simulink library "carnot"  (R2013b)
settings: Solver=ode45  StartTime=0.0  StopTime=10.0  RelTol=1e-3
undefined symbols (not defined in the file or in its folder): A, acol, Ahabit, Awin, Azimuth_Angle, AziWin, B, C, c1, c4, capc, caph, CarnotCallbacks_Density, CarnotCallbacks_Enthalpy, CarnotCallbacks_Enthalpy2Temperature, CarnotCallbacks_Entropy, CarnotCallbacks_Evaporation_Enthalpy, CarnotCallbacks_GlobalMessageLevel, CarnotCallbacks_Grashof, CarnotCallbacks_Heat_Capacity, CarnotCallbacks_Kinematic_Viscosity, CarnotCallbacks_Prandtl, CarnotCallbacks_Saturation_Property, CarnotCallbacks_Saturation_Temperature, CarnotCallbacks_Saturation_Value_Water, CarnotCallbacks_Specific_Volume, CarnotCallbacks_Thermal_Conductivity, CarnotCallbacks_Vapour_Content, CarnotCallbacks_Vapour_Pressure, con, cond, d, Dd, density, dfin, dia, DiameterLastPiece, DPConstant, dpipe, DPLinear, DPQuadratic, emission_out, fluid, FluidMix, FluidType, FPC, frame, g, GeodeticHeight, Gwin, heat_capacity, hgt, HP, Hroom, ID, inlet, K, l, lin, lpipe ... (+29)
undefined symbols (not defined in the file): c2, c3, c5, c6, cwall, dactive, height, mc, mID, rho, tau, UAneighbour, UAwall, uloss
libraries: carnot x333, simulink x25, simulink_extras x7
(part 5 of 16)

== system carnot/Basic/Weather_and_Sun ==
  Cloudage : Subsystem  mask(cloud index){latitude=51, longitude=-7, longitude0=-30, skytype=high mountain}
      mask prompts: latitude "Latitude [-90;90], north positive"; longitude "Longitude  [-180;180], west positive"; longitude0 "reference longitude (timezone)"; skytype "Sky Type"
      mask help:
      | Calculates the cloud index. The cloud index is the fraction of the sky covered by clouds in [0, 1/8, 2/8, 3/8, ..., 7/8, 1].
      |
      | INPUT VECTOR:
      |  time    : real time or simulation time [s]
      |  Iglob   : global radiation on horizontal surface (W/m²)
      |
      | OUTPUT VECTOR:
      |  cloud  : cloudindex [0;1]
      mask Help: web(fullfile(path_carnot('help'),'Cloudage.html'),'-helpbrowser')
      mask TypeOptions skytype: high mountain | lowland | urban region | industrial zone
  Radiation_Divison : Subsystem  mask(Radiation Division){latitude=51, longitude=-7, longitude0=-30}
      mask prompts: latitude "Latitude [-90;90], north positive"; longitude "Longitude  [-180;180], west positive"; longitude0 "reference longitude (timezone)"
      mask help:
      | Calculates the direct and diffusive radiation on the horizontal surface as parts of the global radiation.
      |
      | INPUT VECTOR:
      |   time      : real time or simulation time  [s]
      |   Iglob     : global radiation on horizontal surface (W/m²)
      |
      | OUTPUT VECTORS:
      |   Idir           : direct radiation (W/m²)
      |   Idfu          : diffusive radiation (W/m²)
      |   SunAngle
      |   Zenith
      |   Azimuth
      mask Help: web(fullfile(path_carnot('help'),'Radiation_Divison.html'),'-helpbrowser')
  Sky_Temperature : Subsystem  mask(Sky Temperature){tskymodel=on}
      mask prompts: tskymodel "Include time correction (cos-term in Berdahl equation)"
      mask help:
      | Calculates the skytemperature. If humidity data is availabe, the model of Berdahl and Martin 1984 for low clouds (1000 m) is used.
      | Without humidity data, the model of Unsworth with corrected parameters of Feist 1994 is chosen.
      | INPUT VECTOR:
      |   tamb : ambient temperature [°C]
      |   hum  : humidity [%]
      |   cloud: index of cloudness [0,1]
      |
      | OUTPUT VECTOR:
      |   tsky : sky temperature [°C]
      |
      | The calculation can also be used in m-files with the skytemperature.m function.
      mask Help: web(fullfile(path_carnot('help'),'Sky_Temperature.html'),'-helpbrowser')
  Solar_Declination_Angle : Subsystem  mask(solar declination angle){}
      mask help:
      | The block calls the function "solar_declination" in the CARNOT Library
      | Carlib where the calculation is effectuated. The function solar_declination
      | may be used in m-files. The carlib function solar_declination is also
      | used by the "solar_declination"-block in CARNOT.
      | The equation was taken from Duffie, Beckmann: Solar Engineering of
      | Thermal Processes, 2006. Orginaly the equation was derived by Spencer
      | (Spencer: Fourier Series Representation of the Position of the Sun,
      |  Search Vol.2(5), page 172 , 1971). The error is below 0.035°.
      mask Help: web(fullfile(path_carnot('help'),'Solar_Declination_Angle.html'),'-helpbrowser')
  Solar_Extraterrestrial_Radiation : Subsystem  mask(solar extraterrestrial radiation){}
      mask help:
      | The block calls the function "extraterrestrial_radiation" in the CARNOT Library
      | Carlib where the calculation is effectuated. The function solar_extraterrestrial
      | may be used in m-files. The carlib function extraterrestrial_radiation is also
      | used by the "solar_extraterrestrial_radiation"-block in CARNOT.
      | The equation was taken from Duffie, Beckmann: Solar Engineering of
      | Thermal Processes, 2006. Orginaly the equation was derived by Spencer
      | (Spencer: Fourier Series Representation of the Position of the Sun,
      |  Search Vol.2(5), page 172 , 1971). The accuracy is +- 0.01 %
      mask Help: web(fullfile(path_carnot('help'),'Solar_Extraterrestrial_Radiation.html'),'-helpbrowser')
  Solar_Hour_Angle : Subsystem  mask(Solar Hour Angle){timezone=-15, longitude=-7}
      mask prompts: timezone "longitude of timezone (GMT = 0, east negative) in degree"; longitude "longitude of location (east negative) in degree"
      mask help:
      | The block calls the function "solar_hour_angle" in the CARNOT Library
      | Carlib where the calculation is effectuated.
      | The equation was taken from Duffie, Beckmann: Solar Engineering of
      | Thermal Processes, 2006.
      mask Help: web(fullfile(path_carnot('help'),'Solar_Hour_Angle.html'),'-helpbrowser')
  Solar_Position : Subsystem  mask(Solar Position){lati=45, longi=0, timezone=0}
      mask prompts: lati "Geographical latitude in degree (North postive)"; longi "Geographical longitude in degree (West postive)"; timezone "Latitude of timezone in degree (West postive)"
      mask help:
      | Calculate the solar postion (Duffie, Beckman: Solar Engineering of Thermal Processes, 2008).
      | Output is:
      mask Help: web(fullfile(path_carnot('help'),'Solar_Position.html'),'-helpbrowser')
      mask Display: disp('sunpos')
  Solar_Time : Subsystem  mask(solar time){timezone=-15, longitude=-7}
      mask prompts: timezone "longitude of timezone (GMT = 0, east negative) in degree"; longitude "longitude of location (east negative) in degree"
      mask help:
      | The block calls the function "solar_time" in the CARNOT Library
      | Carlib where the calculation is effectuated. The function solar_time
      | may be used in m-files as "solartime2legaltime" or "legaltime2solartime".
      | The carlib function solar_time is also used by the "solar_time"-block in CARNOT.
      | The equation was taken from Duffie, Beckmann: Solar Engineering of
      | Thermal Processes, 2006. Orginaly the equation was derived by Spencer
      | (Spencer: Fourier Series Representation of the Position of the Sun,
      |  Search Vol.2(5), page 172 , 1971). The accuracy is +- 0.01 %
      mask Help: web(fullfile(path_carnot('help'),'Solar_Time.html'),'-helpbrowser')
  WDB_Creator : Subsystem  mask(Weather Data Bus Creator){}
      mask help: Create the weather data bus with scalar inputs.
      mask Help: web(fullfile(path_carnot('help'),'WDB_Creator.html'),'-helpbrowser')

== system carnot/Control/Controller_Bang_Bang ==
  Thot : Inport
  Tcold : Inport  Port=2
  Constant : Constant  Value=Tmax
  MinMax : MinMax  Function=max  Inputs=2  SaturateOnIntegerOverflow=on  InputSameDT=on
  Product : Product  OutDataTypeStr=double  SaturateOnIntegerOverflow=on
  Relational Operator : RelationalOperator  Operator=<=  InputSameDT=on
  Relay : Relay  OnSwitchValue=deltaTon  OffSwitchValue=deltaToff
  Sum : Sum  Inputs=-+  SaturateOnIntegerOverflow=on  InputSameDT=on  OutDataTypeStr=Inherit: Same as first input
  control : Outport
  wires:
  Sum/1 -> Relay/1
  Constant/1 -> Relational Operator/2
  Thot/1 -> Sum/2, MinMax/2
  Tcold/1 -> Sum/1, MinMax/1
  MinMax/1 -> Relational Operator/1
  Relay/1 -> Product/1
  Product/1 -> control/1
  Relational Operator/1 -> Product/2

== system carnot/Control/EnergyMeter ==
  note: Shows the power in W and the energy in J gain or loss
      | in a fluid flow (characterised by THB) between the
      | inlet and the outlet of one component.
  THB_out : Inport
  THB_in : Inport  Port=2
  Integrator : Integrator  UpperSaturationLimit=1  LowerSaturationLimit=0
  PowerMeter : carnot/Control/PowerMeter
  energy : Outport
  power : Outport  Port=2
  wires:
  THB_out/1 -> PowerMeter/1
  Integrator/1 -> energy/1
  THB_in/1 -> PowerMeter/2
  PowerMeter/1 -> power/1, Integrator/1

== system carnot/Control/EnergyMeter_HC ==
  note: Shows the power in W and the energy in J gain or loss
      | in a fluid flow (characterised by THV) between the
      | inlet and the outlet of one component.
  THB_out : Inport
  THB_in : Inport  Port=2
  Bus Selector : BusSelector  OutputSignals=Temperature
  Bus Selector1 : BusSelector  OutputSignals=Temperature,MassFlow,Pressure,FluidType,FluidMix
  Heat_Capacity : Reference
  Integrator : Integrator  UpperSaturationLimit=1  LowerSaturationLimit=0
  Integrator1 : Integrator  UpperSaturationLimit=1  LowerSaturationLimit=0
  Product : Product  Inputs=***  SaturateOnIntegerOverflow=on  RndMeth=Zero  InputSameDT=on  OutDataTypeStr=Inherit: Same as first input
  T_ave : Gain  Gain=0.5  SaturateOnIntegerOverflow=on  OutDataTypeStr=Inherit: Same as input  ParamDataTypeStr=Inherit: Same as input
  diff_T : Sum  Inputs=+-  SaturateOnIntegerOverflow=on  InputSameDT=on  OutDataTypeStr=Inherit: Same as first input
  only_negative : Saturate  UpperLimit=0  LowerLimit=-inf
  only_positive : Saturate  UpperLimit=inf  LowerLimit=0
  sum : Sum  SaturateOnIntegerOverflow=on  InputSameDT=on  OutDataTypeStr=Inherit: Same as first input
  heating energy : Outport  InitialOutput=0
  power : Outport  Port=2  InitialOutput=0
  cooling energy : Outport  Port=3  InitialOutput=0
  wires:
  THB_in/1 -> Bus Selector/1
  THB_out/1 -> Bus Selector1/1
  Bus Selector1/1 -> diff_T/1, sum/1  "<Temperature>"
  Bus Selector1/4 -> Heat_Capacity/3  "<FluidType>"
  Bus Selector1/5 -> Heat_Capacity/4  "<FluidMix>"
  Heat_Capacity/1 -> Product/1
  Integrator/1 -> heating energy/1
  Bus Selector1/2 -> Product/2  "<MassFlow>"
  diff_T/1 -> Product/3
  Bus Selector/1 -> diff_T/2, sum/2  "<Temperature>"
  sum/1 -> T_ave/1
  T_ave/1 -> Heat_Capacity/1
  Bus Selector1/3 -> Heat_Capacity/2  "<Pressure>"
  Integrator1/1 -> cooling energy/1
  Product/1 -> power/1, only_negative/1, only_positive/1
  only_negative/1 -> Integrator1/1
  only_positive/1 -> Integrator/1

== system carnot/Control/Massflow_Sensor ==
  THB_in : Inport
  Bus Selector : BusSelector  OutputSignals=MassFlow
  heat capacity : StateSpace  A=-tc  B=tc  D=0  X0=t0
  THB : Outport
  mdot : Outport  Port=2
  wires:
  THB_in/1 -> THB/1, Bus Selector/1
  Bus Selector/1 -> heat capacity/1  "<MassFlow>"
  heat capacity/1 -> mdot/1

== system carnot/Control/Max_Run_Time ==
  In : Inport
  Compare To Zero : simulink/Logic and Bit Operations/Compare To Zero  relop=>  OutDataTypeStr=uint8
  Constant : Constant  Value=-1
  Integrator : Integrator  ExternalReset=rising  InitialCondition=tmaxrun  LimitOutput=on  LowerSaturationLimit=0
  Product : Product  RndMeth=Zero
  Out : Outport
  wires:
  Constant/1 -> Integrator/1
  Integrator/1 -> Compare To Zero/1
  Compare To Zero/1 -> Product/1
  In/1 -> Product/2, Integrator/2
  Product/1 -> Out/1

== system carnot/Control/Min_Run_Time ==
  In : Inport
  Compare To Zero : simulink/Logic and Bit Operations/Compare To Zero  relop=>  OutDataTypeStr=uint8
  Constant : Constant  Value=-1
  Gain : Gain  Gain=mv
  Integrator : Integrator  ExternalReset=rising  InitialCondition=tminrun  LimitOutput=on  LowerSaturationLimit=0
  MinMax : MinMax  Function=max  Inputs=2
  Out : Outport
  wires:
  MinMax/1 -> Out/1
  In/1 -> MinMax/2, Integrator/2
  Compare To Zero/1 -> Gain/1
  Integrator/1 -> Compare To Zero/1
  Constant/1 -> Integrator/1
  Gain/1 -> MinMax/1

== system carnot/Control/Min_Stop_Time ==
  In : Inport
  Compare To Zero : simulink/Logic and Bit Operations/Compare To Zero  relop=<=  OutDataTypeStr=uint8
  Compare To Zero1 : simulink/Logic and Bit Operations/Compare To Zero  relop=<=  OutDataTypeStr=uint8
  Constant : Constant  Value=-1
  Integrator : Integrator  ExternalReset=falling  InitialConditionSource=external  InitialCondition=tminstop  LimitOutput=on  LowerSaturationLimit=0  ShowStatePort=on
  Product : Product  RndMeth=Zero
  Product1 : Product  RndMeth=Zero
  Step : Step  Time=0.1  After=tminstop  SampleTime=0
  Out : Outport
  wires:
  Step/1 -> Integrator/3
  Compare To Zero1/1 -> Product/1
  Integrator/State -> Compare To Zero1/1
  Product/1 -> Integrator/2
  Product1/1 -> Out/1
  In/1 -> Product1/2, Product/2
  Compare To Zero/1 -> Product1/1
  Integrator/1 -> Compare To Zero/1
  Constant/1 -> Integrator/1

== system carnot/Control/PowerMeter ==
  THB_out : Inport
  THB_in : Inport  Port=2
  Bus Selector : BusSelector  OutputSignals=Temperature
  Bus Selector1 : BusSelector  OutputSignals=Temperature,MassFlow,Pressure,FluidType,FluidMix
  Heat_Capacity : carnot/Basic/Material_Properties/Heat_Capacity  VariantControl=CarlibClassic  INPUTARGUMENTS=state variables (classic)  DEBUGLEVEL=DEBUGLEVEL  MAXTOTALWARNINGS=inf  MAXCONSECUTIVEWARNINGS=inf  WRITETOFILE=0  FILENAME='errors.txt'
  Product : Product  Inputs=***  SaturateOnIntegerOverflow=on  InputSameDT=on  OutDataTypeStr=Inherit: Same as first input
  T_ave : Gain  Gain=0.5  SaturateOnIntegerOverflow=on  OutDataTypeStr=Inherit: Same as input  ParamDataTypeStr=Inherit: Same as input
  diff_T : Sum  Inputs=+-  SaturateOnIntegerOverflow=on  InputSameDT=on  OutDataTypeStr=Inherit: Same as first input
  sum : Sum  SaturateOnIntegerOverflow=on  InputSameDT=on  OutDataTypeStr=Inherit: Same as first input
  power : Outport
  wires:
  Bus Selector1/1 -> diff_T/1, sum/1  "<Temperature>"
  Bus Selector1/4 -> Heat_Capacity/3  "<FluidType>"
  Bus Selector1/5 -> Heat_Capacity/4  "<FluidMix>"
  Heat_Capacity/1 -> Product/1
  Product/1 -> power/1
  Bus Selector1/2 -> Product/2  "<MassFlow>"
  diff_T/1 -> Product/3
  THB_in/1 -> Bus Selector/1
  Bus Selector/1 -> diff_T/2, sum/2  "<Temperature>"
  sum/1 -> T_ave/1
  T_ave/1 -> Heat_Capacity/1
  Bus Selector1/3 -> Heat_Capacity/2  "<Pressure>"
  THB_out/1 -> Bus Selector1/1

== system carnot/Control/Solar_Radiation_Sensor ==
  WDB : Inport
  Bus Selector : BusSelector  OutputSignals=Solar_Radiation_direct_surface,Solar_Radiation_diffuse_surface
  Idir+Idfu : Sum  Inputs=2  SaturateOnIntegerOverflow=on  InputSameDT=on  OutDataTypeStr=Inherit: Same as first input
  Iglb : Outport
  wires:
  Bus Selector/1 -> Idir+Idfu/1  "<Solar_Radiation_direct_surface>"
  WDB/1 -> Bus Selector/1
  Idir+Idfu/1 -> Iglb/1
  Bus Selector/2 -> Idir+Idfu/2  "<Solar_Radiation_diffuse_surface>"

== system carnot/Control/Start_Delay ==
  In : Inport
  Compare To Zero : simulink/Logic and Bit Operations/Compare To Zero  relop=<=  OutDataTypeStr=uint8
  Constant : Constant  Value=-1
  Integrator : Integrator  ExternalReset=rising  InitialCondition=tstartdelay  LimitOutput=on  LowerSaturationLimit=0
  Product1 : Product  RndMeth=Zero
  Out : Outport
  wires:
  Constant/1 -> Integrator/1
  Integrator/1 -> Compare To Zero/1
  Compare To Zero/1 -> Product1/1
  In/1 -> Product1/2, Integrator/2
  Product1/1 -> Out/1

== system carnot/Control/T_Sensor ==
  THB_in : Inport
  Bus Selector : BusSelector  OutputSignals=Temperature
  heat capacity : StateSpace  A=-tc  B=tc  D=0  X0=t0
  THB : Outport
  T : Outport  Port=2
  wires:
  THB_in/1 -> THB/1, Bus Selector/1
  Bus Selector/1 -> heat capacity/1  "<Temperature>"
  heat capacity/1 -> T/1

== system carnot/Control/T_Sensor_Surface ==
  note: sensor_node = max(ceil(position*nodes),1)
  Tnodes : Inport
  Constant : Constant  Value=ones(length(pos),1)
  Gain : Gain  Gain=pos  Multiplication=Matrix(u*K)
  Gain1 : Gain  Gain=1/tdel
  Integrator : Integrator  InitialCondition=t0
  MinMax : MinMax  Function=max  Inputs=2
  Rounding Function : Rounding  Operator=ceil
  Selector : Selector  IndexOptions=Index vector (port)  Indices=[1 3]  OutputSizes=1
  Sum : Sum  Inputs=|+-
  Width : Width
  Tsurf : Outport
  wires:
  MinMax/1 -> Selector/2
  Constant/1 -> MinMax/2
  Rounding Function/1 -> MinMax/1
  Gain/1 -> Rounding Function/1
  Selector/1 -> Sum/1
  Integrator/1 -> Tsurf/1, Sum/2
  Sum/1 -> Gain1/1
  Tnodes/1 -> Selector/1, Width/1
  Width/1 -> Gain/1
  Gain1/1 -> Integrator/1

== system carnot/Control/Window_Control ==
  Tamb : Inport
  Troom : Inport  Port=2
  24h Moving Average : DiscreteFir  Coefficients=ones(1,24)*(1/24)  SampleTime=3600  AccumDataTypeStr=Inherit: Same as product output  RndMeth=Nearest
  Clock2 : Clock
  Direct Lookup Table (n-D) : LookupNDDirect  NumberOfTableDimensions=1  Table=[0 1]
  J->kWh7 : Gain  Gain=1/3600  SaturateOnIntegerOverflow=on  OutDataTypeStr=Inherit: Same as input  ParamDataTypeStr=Inherit: Same as input
  Logical Operator : Logic  Operator=OR  AllPortsSameDT=off  OutDataTypeStr=boolean
  Logical Operator1 : Logic  Inputs=3  AllPortsSameDT=off  OutDataTypeStr=boolean
  Math Function : Math  Operator=rem  SaturateOnIntegerOverflow=on
  Product : Product  RndMeth=Zero
  Relational Operator : RelationalOperator  Operator=<=  OutDataTypeStr=boolean
  Relational Operator1 : RelationalOperator  Operator=<=  OutDataTypeStr=boolean
  Relational Operator2 : RelationalOperator  Operator=<=  OutDataTypeStr=boolean
  Relay : Relay  OnSwitchValue=24  OffSwitchValue=23
  Rounding Function : Rounding
  Subtract : Sum  Inputs=+-
  const1 : Constant  Value=24*3600
  const2 : Constant  Value=8
  const3 : Constant  Value=21
  const4 : Constant  Value=12
  const6 : Constant  Value=2
  op2 : RelationalOperator  Operator=<=  OutDataTypeStr=boolean
  control : Outport
  wires:
  Clock2/1 -> Math Function/1
  const1/1 -> Math Function/2
  Math Function/1 -> J->kWh7/1
  J->kWh7/1 -> Rounding Function/1
  Rounding Function/1 -> Relational Operator/1, Relational Operator1/2
  const2/1 -> Relational Operator/2
  const3/1 -> Relational Operator1/1
  Relational Operator1/1 -> Logical Operator/1
  Relational Operator/1 -> Logical Operator/2
  Tamb/1 -> Subtract/2, 24h Moving Average/1
  const4/1 -> op2/1
  Logical Operator/1 -> Logical Operator1/3
  Troom/1 -> Relay/1, Subtract/1  "room temperature [°C]"
  const6/1 -> Relational Operator2/1
  Subtract/1 -> Relational Operator2/2
  Relational Operator2/1 -> Logical Operator1/1
  Logical Operator1/1 -> Direct Lookup Table (n-D)/1
  op2/1 -> Logical Operator1/2
  Direct Lookup Table (n-D)/1 -> Product/2
  Product/1 -> control/1
  Relay/1 -> Product/1
  24h Moving Average/1 -> op2/2

== system carnot/Hydraulics/Flow_Diverter ==
  THB : Inport
  fdiv : Inport  Port=2
  Bus Assignment : BusAssignment  AssignedSignals=ID,MassFlow,DPConstant,DPLinear,DPQuadratic
  Bus Assignment1 : BusAssignment  AssignedSignals=ID,MassFlow,DPConstant,DPLinear,DPQuadratic
  Bus Selector : BusSelector  OutputSignals=MassFlow
  Bus Selector4 : BusSelector  OutputSignals=ID
  Dot Product : DotProduct  InputSameDT=on  OutDataTypeStr=Inherit: Inherit via internal rule
  Saturation : Saturate  UpperLimit=1  LowerLimit=0
  Subsystem : Subsystem
  Sum : Sum  Inputs=-+  SaturateOnIntegerOverflow=on  InputSameDT=on  OutDataTypeStr=Inherit: Same as first input
  const{,1..2,4..6} (6 alike) : Constant  Value=0
  increase_ID : Subsystem
  THB1 : Outport
  THB2 : Outport  Port=2
  clq : Outport  Port=3
  wires:
  Subsystem/1(Out1) -> clq/1
  Bus Assignment1/1 -> THB2/1
  Bus Assignment/1 -> THB1/1
  const4/1 -> Bus Assignment/4  "DPConstant"
  const5/1 -> Bus Assignment/5  "DPLinear"
  const6/1 -> Bus Assignment/6  "DPQuadratic"
  increase_ID/1(Out1) -> Bus Assignment1/2, Bus Assignment/2  "ID"
  Bus Selector4/1 -> increase_ID/1(In1)  "<ID>"
  Dot Product/1 -> Bus Assignment/3, Sum/1  "MassFlow"
  fdiv/1 -> Saturation/1
  THB/1 -> Subsystem/1(In1), Bus Assignment1/1, Bus Selector4/1, Bus Assignment/1, Bus Selector/1
  const/1 -> Bus Assignment1/4  "DPConstant"
  Bus Selector/1 -> Sum/2, Dot Product/1  "<MassFlow>"
  Sum/1 -> Bus Assignment1/3  "MassFlow"
  Saturation/1 -> Dot Product/2
  const1/1 -> Bus Assignment1/5  "DPLinear"
  const2/1 -> Bus Assignment1/6  "DPQuadratic"

== system carnot/Hydraulics/Flow_Mixer ==
  THB1 : Inport
  THB2 : Inport  Port=2
  clq : Inport  Port=3
  Flow_Mixer_basic : carnot/Basic/Hydraulics/Flow_Mixer_basic
  PT1_for_fdiv : Subsystem
  THB : Outport
  fdiv : Outport  Port=2
  wires:
  Flow_Mixer_basic/4 -> PT1_for_fdiv/3(fdiv)
  Flow_Mixer_basic/3 -> PT1_for_fdiv/2(ID_2)
  Flow_Mixer_basic/2 -> PT1_for_fdiv/1(ID_1)
  Flow_Mixer_basic/1 -> THB/1
  THB2/1 -> Flow_Mixer_basic/2
  THB1/1 -> Flow_Mixer_basic/1
  PT1_for_fdiv/1(f_div) -> fdiv/1
  clq/1 -> Flow_Mixer_basic/3

== system carnot/Hydraulics/Flow_Mixer_Thermostatic ==
  THBhot : Inport
  THBcold : Inport  Port=2
  clq : Inport  Port=3
  Tset : Inport  Port=4
  Bus Selector : BusSelector  OutputSignals=Temperature
  Flow_Mixer_basic : carnot/Basic/Hydraulics/Flow_Mixer_basic
  Icontrol_fdiv : Subsystem
  Terminator : Terminator
  THB : Outport
  fdiv : Outport  Port=2
  wires:
  Bus Selector/1 -> Icontrol_fdiv/3(Twarm)  "<Temperature>"
  Flow_Mixer_basic/4 -> Terminator/1
  Tset/1 -> Icontrol_fdiv/4(Tset)
  Flow_Mixer_basic/3 -> Icontrol_fdiv/2(ID_2)
  Flow_Mixer_basic/2 -> Icontrol_fdiv/1(ID_1)
  Flow_Mixer_basic/1 -> Bus Selector/1, THB/1
  clq/1 -> Flow_Mixer_basic/3
  THBcold/1 -> Flow_Mixer_basic/2
  THBhot/1 -> Flow_Mixer_basic/1
  Icontrol_fdiv/1(f_div) -> fdiv/1

== system carnot/Hydraulics/Pipe ==
  Tamb : Inport
  THBin : Inport  Port=2
  Constant : Constant  Value=hgt
  Pipe_basic : carnot/Basic/Thermal_Models/Pipe_basic  vol=pi*(dia/2)^2*len  L=len  uloss=uloss  effcond=cond  cwall=cwall  t0=t0  nodes=nodes
  Pressure_Drop_Fix : carnot/Basic/Pressure_Drop/Pressure_Drop_Fix  con=0  lin=lin  qua=qua
  Pressure_Drop_changeD : carnot/Basic/Pressure_Drop/Pressure_Drop_changeD  dia=dia
  Pressure_Drop_staticHeight : carnot/Basic/Pressure_Drop/Pressure_Drop_staticHeight
  THB : Outport
  wires:
  Pipe_basic/2 -> Pressure_Drop_staticHeight/2
  Pipe_basic/1 -> Pressure_Drop_staticHeight/1
  Tamb/1 -> Pipe_basic/1
  THBin/1 -> Pipe_basic/2
  Constant/1 -> Pressure_Drop_staticHeight/3
  Pressure_Drop_staticHeight/1 -> Pressure_Drop_Fix/1
  Pressure_Drop_Fix/1 -> Pressure_Drop_changeD/1
  Pressure_Drop_changeD/1 -> THB/1

== system carnot/Hydraulics/Pipe_Geometry ==
  Tamb : Inport
  THBin : Inport  Port=2
  Constant : Constant  Value=hgt
  Pipe_basic : carnot/Basic/Thermal_Models/Pipe_basic  vol=pi*(dia/2)^2*len  L=len  uloss=uloss  effcond=cond  cwall=cwall  t0=t0  nodes=nodes
  Pressure_Drop_PipeTheory : carnot/Basic/Pressure_Drop/Pressure_Drop_PipeTheory  dia=dia  len=len  rough=rough  nbend=nbend
  Pressure_Drop_changeD : carnot/Basic/Pressure_Drop/Pressure_Drop_changeD  dia=dia
  Pressure_Drop_staticHeight : carnot/Basic/Pressure_Drop/Pressure_Drop_staticHeight
  THB : Outport
  wires:
  Pressure_Drop_PipeTheory/1 -> Pressure_Drop_changeD/1
  Pressure_Drop_staticHeight/1 -> Pressure_Drop_PipeTheory/2
  Pressure_Drop_changeD/1 -> THB/1
  Constant/1 -> Pressure_Drop_staticHeight/3
  Pipe_basic/2 -> Pressure_Drop_staticHeight/2
  Pipe_basic/1 -> Pressure_Drop_PipeTheory/1, Pressure_Drop_staticHeight/1
  THBin/1 -> Pipe_basic/2
  Tamb/1 -> Pipe_basic/1

== system carnot/Hydraulics/Pipe_Isolation ==
  Tamb : Inport
  THBin : Inport  Port=2
  Constant : Constant  Value=hgt
  Pipe_basic : carnot/Basic/Thermal_Models/Pipe_basic  vol=pi*(dia/2)^2*len  L=len  uloss=uloss  effcond=cond  cwall=cwall  t0=t0  nodes=nodes
  Pressure_Drop_Fix : carnot/Basic/Pressure_Drop/Pressure_Drop_Fix  con=0  lin=lin  qua=qua
  Pressure_Drop_changeD : carnot/Basic/Pressure_Drop/Pressure_Drop_changeD  dia=dia
  Pressure_Drop_staticHeight : carnot/Basic/Pressure_Drop/Pressure_Drop_staticHeight
  THB : Outport
  wires:
  Pipe_basic/2 -> Pressure_Drop_staticHeight/2
  Pipe_basic/1 -> Pressure_Drop_staticHeight/1
  Pressure_Drop_changeD/1 -> THB/1
  Pressure_Drop_Fix/1 -> Pressure_Drop_changeD/1
  Pressure_Drop_staticHeight/1 -> Pressure_Drop_Fix/1
  Constant/1 -> Pressure_Drop_staticHeight/3
  THBin/1 -> Pipe_basic/2
  Tamb/1 -> Pipe_basic/1

== system carnot/Hydraulics/Pump_Additional ==
  THBin : Inport
  control : Inport  Port=2
  Abs : Abs
  Bus Assignment : BusAssignment  AssignedSignals=ID,Temperature,Pressure,DiameterLastPiece,DPConstant,DPLinear,DPQuadratic
  Bus Selector : BusSelector  OutputSignals=Temperature,MassFlow
  Bus Selector1 : BusSelector  OutputSignals=ID
  Bus Selector2 : BusSelector  OutputSignals=MassFlow
  Bus Selector3 : BusSelector  OutputSignals=DPConstant,DPLinear,DPQuadratic  OutputAsBus=on
  Bus Selector5 : BusSelector  OutputSignals=MassFlow
  Bus Selector6 : BusSelector  OutputSignals=Pressure
  Constant : Constant  Value=dia
  Constant1 : Constant  Value=-a1
  Constant2 : Constant  Value=-a2
  Demux : Demux  Outputs=3
  Density : carnot/Basic/Material_Properties/Density  VariantControl=CarlibClassic  INPUTARGUMENTS=THB  DEBUGLEVEL=DEBUGLEVEL  MAXTOTALWARNINGS=inf  MAXCONSECUTIVEWARNINGS=inf  WRITETOFILE=0  FILENAME='errors.txt'
  Gain : Gain  Gain=-a0
  Pressuredrop : carnot/Basic/Pressure_Drop/Pressuredrop
  Product : Product  Inputs=**//  SaturateOnIntegerOverflow=on  InputSameDT=on  OutDataTypeStr=Inherit: Same as first input
  Saturation : Saturate  UpperLimit=1  LowerLimit=0
  Switch3 : Switch  Criteria=u2 > Threshold  SaturateOnIntegerOverflow=on  InputSameDT=on
  Thermal_Capacity : carnot/Basic/Thermal_Models/Thermal_Capacity  UA=1  mcp=t1*100  Tamb=20  cp_approx=4000
  gain1 : Gain  Gain=-1  SaturateOnIntegerOverflow=on  OutDataTypeStr=Inherit: Same as input  ParamDataTypeStr=Inherit: Same as input
  pump efficiency : Lookup  InputValues=0:1:5  Table=[0.001 0.5 0.7 0.7 0.5 0.001]  SaturateOnIntegerOverflow=on
  THB : Outport
  Power : Outport  Port=2
  wires:
  Demux/3 -> Bus Assignment/8
  Demux/2 -> Bus Assignment/7
  Demux/1 -> Bus Assignment/6
  Pressuredrop/2 -> Demux/1
  Constant2/1 -> Pressuredrop/6
  Constant1/1 -> Pressuredrop/5
  Gain/1 -> Pressuredrop/4
  Bus Selector3/1 -> Pressuredrop/3
  Constant/1 -> Bus Assignment/5
  Pressuredrop/1 -> Bus Assignment/4
  Bus Assignment/1 -> THB/1
  Bus Selector6/1 -> Pressuredrop/2  "<Pressure>"
  Bus Selector5/1 -> Pressuredrop/1  "<MassFlow>"
  Pressuredrop/3 -> Product/2
  Switch3/1 -> Bus Assignment/2  "ID"
  gain1/1 -> Switch3/3
  Abs/1 -> gain1/1
  Bus Selector1/1 -> Abs/1, Switch3/1  "<ID>"
  Saturation/1 -> Gain/1, Switch3/2
  Bus Selector2/1 -> pump efficiency/1, Product/1  "<MassFlow>"
  Bus Selector/2 -> Thermal_Capacity/2  "<MassFlow>"
  Bus Selector/1 -> Thermal_Capacity/1  "<Temperature>"
  Product/1 -> Power/1
  THBin/1 -> Bus Assignment/1, Bus Selector2/1, Density/1, Bus Selector3/1, Bus Selector6/1, Bus Selector5/1, Bus Selector1/1, Bus Selector/1
  pump efficiency/1 -> Product/3
  Density/1 -> Product/4
  control/1 -> Saturation/1
  Thermal_Capacity/1 -> Bus Assignment/3  "T"

== system carnot/Hydraulics/Pump_Const ==
  THBin : Inport
  control : Inport  Port=2
  Bus Assignment : BusAssignment  AssignedSignals=Temperature
  Bus Selector : BusSelector  OutputSignals=Temperature,MassFlow
  Pump_basic : carnot/Basic/Hydraulics/Pump_basic  mdotmax=mdotmax  fluid_id=fluid_id  mix=mix  dia=dia  power=power  p0=p0  hgt=0  ID=1
  Thermal_Capacity : carnot/Basic/Thermal_Models/Thermal_Capacity  UA=UA  mcp=mcp  Tamb=tamb  cp_approx=4000
  THB : Outport
  power : Outport  Port=2
  wires:
  Pump_basic/1 -> Bus Assignment/1, Bus Selector/1
  THBin/1 -> Pump_basic/1
  Bus Selector/1 -> Thermal_Capacity/1  "<Temperature>"
  Thermal_Capacity/1 -> Bus Assignment/2  "T"
  control/1 -> Pump_basic/2
  Bus Selector/2 -> Thermal_Capacity/2  "<MassFlow>"
  Pump_basic/2 -> power/1
  Bus Assignment/1 -> THB/1

== system carnot/Hydraulics/Pump_Main ==
  THBin : Inport
  control : Inport  Port=2
  Bus Assignment : BusAssignment  AssignedSignals=ID,Temperature,MassFlow
  Bus Selector : BusSelector  OutputSignals=ID,Temperature,MassFlow,Pressure
  Bus Selector1 : BusSelector  OutputSignals=DPConstant,DPLinear,DPQuadratic  OutputAsBus=on
  Density : carnot/Basic/Material_Properties/Density  VariantControl=CarlibClassic  INPUTARGUMENTS=THB  DEBUGLEVEL=DEBUGLEVEL  MAXTOTALWARNINGS=inf  MAXCONSECUTIVEWARNINGS=inf  WRITETOFILE=0  FILENAME='errors.txt'
  Gain : Gain  Gain=a0
  ID : Constant  Value=ID
  Mux2 : Mux  Inputs=5
  Product : Product  Inputs=**//  SaturateOnIntegerOverflow=on  InputSameDT=on  OutDataTypeStr=Inherit: Same as first input
  S-Function : S-Function  FunctionName=pump  EnableBusSupport=off
  Sum : Sum  Inputs=-+
  Switch1 : Switch  Criteria=u2 > Threshold  SaturateOnIntegerOverflow=on  InputSameDT=on
  Switch3 : Switch  Criteria=u2 > Threshold  SaturateOnIntegerOverflow=on  InputSameDT=on
  Transfer Fcn (with initial states) : simulink_extras/Additional Linear/Transfer Fcn (with initial states)  N=[1]  D="[t1  1]"  X0=0
  basic_THB : carnot/Basic/Hydraulics/basic_THB  t=20  mdot=0  p=p0  ID=ID  fluid=fluid_id  mix=mix  dia=dia  hgt=0
  const2 : Constant  Value=p0
  const3 : Constant  Value=a1
  const4 : Constant  Value=a2
  const5 : Constant  Value=0
  gain1 : Gain  Gain=-1  SaturateOnIntegerOverflow=on  OutDataTypeStr=Inherit: Same as input  ParamDataTypeStr=Inherit: Same as input
  pump efficiency : Lookup  InputValues=0:1:5  Table=[0.001 0.5 0.7 0.7 0.5 0.001]  SaturateOnIntegerOverflow=on
  thermal_capacity : carnot/Basic/Thermal_Models/Thermal_Capacity  UA=ua  mcp=mcp  Tamb=tamb  cp_approx=4000
  THB : Outport
  Power : Outport  Port=2
  wires:
  Bus Selector1/1 -> Mux2/2  "clq"
  THBin/1 -> Bus Selector/1, Bus Selector1/1, Density/1
  Switch1/1 -> Bus Assignment/4
  thermal_capacity/1 -> Bus Assignment/3
  Switch3/1 -> Bus Assignment/2
  Bus Assignment/1 -> THB/1
  basic_THB/1 -> Bus Assignment/1
  const5/1 -> Switch1/3
  Transfer Fcn (with initial states)/1 -> Switch1/1
  gain1/1 -> Switch3/3
  ID/1 -> Switch3/1, gain1/1
  control/1 -> Switch3/2, Gain/1
  Gain/1 -> Mux2/3
  const4/1 -> Mux2/5
  const3/1 -> Mux2/4
  S-Function/1 -> Transfer Fcn (with initial states)/1
  Density/1 -> Product/4
  pump efficiency/1 -> Product/3
  Mux2/1 -> S-Function/1
  Bus Selector/2 -> thermal_capacity/1  "<Temperature>"
  Bus Selector/3 -> thermal_capacity/2, Product/1, pump efficiency/1  "<MassFlow>"
  Bus Selector/4 -> Sum/1  "<Pressure>"
  Bus Selector/1 -> Switch1/2, Mux2/1  "<ID>"
  Product/1 -> Power/1
  Sum/1 -> Product/2
  const2/1 -> Sum/2

== system carnot/Hydraulics/Pump_Simple ==
  THBin : Inport
  control : Inport  Port=2
  Pump_basic : carnot/Basic/Hydraulics/Pump_basic  mdotmax=mdotmax  fluid_id=fluid_id  mix=mix  dia=dia  power=power  p0=p0  hgt=0  ID=1
  THB : Outport
  power : Outport  Port=2
  wires:
  THBin/1 -> Pump_basic/1
  control/1 -> Pump_basic/2
  Pump_basic/1 -> THB/1
  Pump_basic/2 -> power/1

== system carnot/Hydraulics/Thermosyphon ==
  THBin : Inport
  Bus Assignment : BusAssignment  AssignedSignals=Temperature,MassFlow
  Bus Selector : BusSelector  OutputSignals=Temperature,MassFlow
  Bus Selector1 : BusSelector  OutputSignals=DPConstant,DPLinear,DPQuadratic  OutputAsBus=on
  Bus Selector2 : BusSelector  OutputSignals=ID
  Bus Selector3 : BusSelector  OutputSignals=GeodeticHeight  OutputAsBus=on
  Check difference in height : simulink/Model Verification/Check  Static Range  Description=-0.001 <= u <= 0.001  max=0.001  max_included=on  min=-0.001  min_included=on  enabled=on  stopWhenAssertionFail=on  export=off  icon=graphic
  Mux2 : Mux  Inputs=5
  S-Function : S-Function  FunctionName=pump  EnableBusSupport=off
  Switch1 : Switch  Criteria=u2 > Threshold  SaturateOnIntegerOverflow=on  InputSameDT=on
  Transfer Fcn (with initial states) : simulink_extras/Additional Linear/Transfer Fcn (with initial states)  N=[1]  D="[t1  1]"  X0=0
  basic_THB : carnot/Basic/Hydraulics/basic_THB  t=20  mdot=0  p=p0  ID=20001  fluid=fluid_id  mix=mix  dia=dia  hgt=0
  const{1,3..5} (4 alike) : Constant  Value=0
  thermal_capacity : carnot/Basic/Thermal_Models/Thermal_Capacity  UA=1  mcp=t1*100  Tamb=20  cp_approx=4000
  THB : Outport
  wires:
  Bus Selector3/1 -> Check difference in height/1
  Switch1/1 -> Bus Assignment/3
  thermal_capacity/1 -> Bus Assignment/2
  Bus Selector1/1 -> Mux2/2  "clq"
  Bus Assignment/1 -> THB/1
  basic_THB/1 -> Bus Assignment/1
  const5/1 -> Switch1/3
  Transfer Fcn (with initial states)/1 -> Switch1/1
  const1/1 -> Mux2/3
  const4/1 -> Mux2/5
  const3/1 -> Mux2/4
  S-Function/1 -> Transfer Fcn (with initial states)/1
  Mux2/1 -> S-Function/1
  Bus Selector/1 -> thermal_capacity/1  "<Temperature>"
  Bus Selector/2 -> thermal_capacity/2  "<MassFlow>"
  Bus Selector2/1 -> Switch1/2, Mux2/1  "<ID>"
  THBin/1 -> Bus Selector3/1, Bus Selector1/1, Bus Selector2/1, Bus Selector/1

== system carnot/Hydraulics/Valve ==
  THBin : Inport
  position : Inport  Port=2
  Abs : Abs
  Bus Assignment : BusAssignment  AssignedSignals=ID,Pressure,DPConstant,DPLinear,DPQuadratic
  Bus Selector : BusSelector  OutputSignals=ID,MassFlow,Pressure
  Bus Selector1 : BusSelector  OutputSignals=DPConstant,DPLinear,DPQuadratic  OutputAsBus=on
  Constant : Constant  Value=0
  Constant1 : Constant  Value=0
  Demux : Demux  Outputs=3
  Saturation : Saturate  UpperLimit=1  LowerLimit=0
  Switch1 : Switch  Criteria=u2 > Threshold  SaturateOnIntegerOverflow=on  InputSameDT=on
  Terminator : Terminator
  gain2 : Gain  Gain=-1  SaturateOnIntegerOverflow=on  OutDataTypeStr=Inherit: Same as input  ParamDataTypeStr=Inherit: Same as input
  pressuredrop : carnot/Basic/Pressure_Drop/Pressuredrop
  valve characteristic : Lookup  InputValues=pos_values  Table=dp_values  SaturateOnIntegerOverflow=on
  THB : Outport
  wires:
  Demux/3 -> Bus Assignment/6
  Demux/2 -> Bus Assignment/5
  Demux/1 -> Bus Assignment/4
  Bus Assignment/1 -> THB/1
  THBin/1 -> Bus Assignment/1, Bus Selector1/1, Bus Selector/1
  pressuredrop/3 -> Terminator/1
  valve characteristic/1 -> pressuredrop/6
  Constant1/1 -> pressuredrop/5
  Constant/1 -> pressuredrop/4
  pressuredrop/2 -> Demux/1  "clq"
  Bus Selector/3 -> pressuredrop/2  "<Pressure>"
  Abs/1 -> gain2/1
  Switch1/1 -> Bus Assignment/2  "ID"
  Saturation/1 -> valve characteristic/1
  Bus Selector/2 -> pressuredrop/1  "<MassFlow>"
  pressuredrop/1 -> Bus Assignment/3  "p"
  Bus Selector1/1 -> pressuredrop/3  "clq"
  position/1 -> Saturation/1, Switch1/2
  Bus Selector/1 -> Abs/1, Switch1/1  "<ID>"
  gain2/1 -> Switch1/3

== system carnot/Hydraulics/Valve_ThermoTset ==
  THB_in : Inport
  Troom : Inport  Port=2
  Tset : Inport  Port=3
  Valve : carnot/Hydraulics/Valve  pos_values=vpos  dp_values=vqua
  thermostat charcteristic : Subsystem
  THB_out : Outport
  wires:
  Troom/1 -> thermostat charcteristic/1(T)
  Tset/1 -> thermostat charcteristic/2(Tset)
  THB_in/1 -> Valve/1
  Valve/1 -> THB_out/1
  thermostat charcteristic/1(pos) -> Valve/2

== system carnot/Hydraulics/Valve_ThermoTset_fn ==
  THB : Inport
  Troom : Inport  Port=2
  Tset : Inport  Port=3
  Valve_fn : carnot/Hydraulics/Valve_fn  kv=kv  kvs=kvs  op=op
  thermostat charcteristic : carnot/Hydraulics/Valve_ThermoTset/thermostat charcteristic
  THB_out : Outport  InitialOutput=0
  pos : Outport  Port=2  InitialOutput=0
  wires:
  thermostat charcteristic/1 -> Valve_fn/2, pos/1
  THB/1 -> Valve_fn/1
  Tset/1 -> thermostat charcteristic/2
  Troom/1 -> thermostat charcteristic/1
  Valve_fn/1 -> THB_out/1

== system carnot/Hydraulics/Valve_Thermostatic ==
  THBin : Inport
  Troom : Inport  Port=2
  Valve_ThermoTset : carnot/Hydraulics/Valve_ThermoTset  p=prange  op=op  bl=bl  ts=ts  dia=dia  vpos=vpos  vqua=vqua
  offset : Constant  Value=Tset
  THB : Outport
  wires:
  offset/1 -> Valve_ThermoTset/3
  Troom/1 -> Valve_ThermoTset/2
  THBin/1 -> Valve_ThermoTset/1
  Valve_ThermoTset/1 -> THB/1

== system carnot/Hydraulics/Valve_fn ==
  note: 2.8e6*(0.685/(0.9*(2/(1+exp(-2/op*u(1)))-1)))^2
      | 2.8e6*(kv/(kvs*(2/(1+exp(-2/op*u(1)))-1)))^2
      |
      | char = kv/(kvs*(2/(1+exp(-2/op*u(1)))-1))
      | res = 2.8e6*(char)^2
  THBin : Inport
  position : Inport  Port=2
  Abs : Abs
  Bus Assignment : BusAssignment  AssignedSignals=ID,Pressure,DPConstant,DPLinear,DPQuadratic
  Bus Selector : BusSelector  OutputSignals=ID,MassFlow,Pressure
  Bus Selector1 : BusSelector  OutputSignals=DPConstant,DPLinear,DPQuadratic  OutputAsBus=on
  Constant : Constant  Value=0
  Constant1 : Constant  Value=0
  Demux : Demux  Outputs=3
  Fcn_data : Fcn  Expr=2.8e6*(kv/(kvs*(2/(1+exp(-2/op*u(1)))-1)))^2
  Saturation : Saturate  UpperLimit=1  LowerLimit=1e-9
  Switch1 : Switch  Criteria=u2 > Threshold  SaturateOnIntegerOverflow=on  InputSameDT=on
  Terminator : Terminator
  gain2 : Gain  Gain=-1  SaturateOnIntegerOverflow=on  OutDataTypeStr=Inherit: Same as input  ParamDataTypeStr=Inherit: Same as input
  pressuredrop : carnot/Basic/Pressure_Drop/Pressuredrop
  THB : Outport  InitialOutput=0
  wires:
  gain2/1 -> Switch1/3
  Bus Selector/1 -> Switch1/1, Abs/1  "<ID>"
  position/1 -> Saturation/1, Switch1/2
  Bus Selector1/1 -> pressuredrop/3  "clq"
  pressuredrop/1 -> Bus Assignment/3  "p"
  Bus Selector/2 -> pressuredrop/1  "<MassFlow>"
  Switch1/1 -> Bus Assignment/2  "ID"
  Abs/1 -> gain2/1
  Bus Selector/3 -> pressuredrop/2  "<Pressure>"
  pressuredrop/2 -> Demux/1  "clq"
  Constant/1 -> pressuredrop/4
  Constant1/1 -> pressuredrop/5
  pressuredrop/3 -> Terminator/1
  THBin/1 -> Bus Selector/1, Bus Selector1/1, Bus Assignment/1
  Bus Assignment/1 -> THB/1
  Demux/1 -> Bus Assignment/4
  Demux/2 -> Bus Assignment/5
  Demux/3 -> Bus Assignment/6
  Fcn_data/1 -> pressuredrop/6
  Saturation/1 -> Fcn_data/1

== system carnot/Load/General ==
  Load_Data_Button : Subsystem
      settings: OpenFcn=|
      | [filename, pathname, filterindex] = ...
      |    uigetfile( {'*.mat','MAT-files (*.mat)'; ...
      |    '*.*',  'All Files (*.*)'},  'Pick a data file');
      | 
      | if (filterindex > 0)
      |    load(filename)
      | end
      mask Display: disp('double click \nto load data')
  Load_from_File : Subsystem  mask(Load from File){file=FileName, ext=.mat}
      mask prompts: file "Name of file"; ext "Extension of file"
      mask help:
      | Input block for external load data files. The file is read to the workspace. A "From Workspace" Block is used in the subsystem.
      | A Unit-Delay with the timestep of the data forces the model to a maximum timestep equal to the data acquisiton timestep.
      mask init:
      | parampath = '';
      | CarnotCallbacks_GetFiles;
      | 
      | %if evalin('base',['exist (''' filename ext ''',''file'');'])
      | %    evalin('base',[filename '= importdata(''' filename ext ''');']);
      | %end
      | % set_param([gcb '/Data_from_Workspace'], 'VariableName', filename);
      | % sample time is timestep of weather data
      | % evalin('caller',['t_sample = ' filename '(3,1) - ' filename '(2,1);']);
      mask Help: web(fullfile(path_carnot('help'),'Load_from_file.html'),'-helpbrowser')
      mask TypeOptions ext: .dat | .txt | .mat
      mask Display: disp(file)
  Repeating_Profile : Subsystem  mask(Repeating Profile){period=24*3600, rep_seq_t=[0 6 7 8 9 11 12 13 14 15 17 18 20 21 22]*3600, rep_seq_d=[6 1 1 1 2 1 1 1 1 2 1 2 1 1 2]*3600, rep_seq_y=[4 2 3 2 0 1 3 2 1 0 1 2 4 3 4]*60}
      mask prompts: period "Time period in s"; rep_seq_t "Time values in s"; rep_seq_d "Duration in s"; rep_seq_y "Output values:"
      mask help:
      | Repeating load profile. The period must be larger than the last time value and the time values must be monotonically ingreasing.
      | Duration is a vector with the same number of elements than the time values. Each duration corresponts to one time value.
      | The number of output values must be the same as the number of time values. Each output value corresponds to one time value.
      mask init:
      | if (length(rep_seq_t) ~= length(rep_seq_y)),
      |   error('Length of time vector and output vector must be the same.')
      | elseif (max(rep_seq_t) > period)
      |   error('Time period must be larger than last time value')
      | end
      | 
      | disp_t1 = rep_seq_t'*[1 1];
      | disp_t2 = (rep_seq_t+rep_seq_d)'*[1 1];
      | disp_t = [disp_t1 disp_t2]';
      | disp_t = [0 reshape(disp_t,1,prod(size(disp_t))) period];
      | 
      | disp_y = rep_seq_y'*[1 1 0 0];
      | disp_y = [0 0 reshape(disp_y',1,prod(size(disp_y)))];
      mask Help: web(fullfile(path_carnot('help'),'Repeating_Profile.html'),'-helpbrowser')
      mask Display: plot( disp_t, disp_y )
